simulink model "push_set_reset_Codegen"  (R2021a)
settings: Solver=FixedStepDiscrete  StartTime=0.0  StopTime=10  RelTol=1e-3
libraries: simulink x1
settings Model: Creator=surya  LastModifiedBy=surya
settings OptimizationCC: DefaultParameterBehavior=Inlined  EnhancedBackFolding=on  PassReuseOutputArgsAs=Individual arguments  ZeroExternalMemoryAtStartup=off  ZeroInternalMemoryAtStartup=off  OptimizeBlockOrder=speed  DifferentSizesBufferReuse=on  OptimizationCustomize=off  EfficientTunableParamExpr=on
settings DebuggingCC: ParameterTunabilityLossMsg=error
settings SFSimCC: MATLABDynamicMemAlloc=off
settings RTWCC: SystemTargetFile=ert.tlc  TemplateMakefile=ert_default_tmf
settings CodeAppCC: ForceParamTrailComments=on  IgnoreCustomStorageClasses=off  OperatorAnnotations=on  SimulinkDataObjDesc=on  SFDataObjDesc=on  InsertBlockDesc=on
settings ERTTargetCC: TargetLangStandard=C99 (ISO)  GenerateSampleERTMain=on  InlinedParameterPlacement=NonHierarchical  ERTCustomFileTemplate=example_file_process.tlc

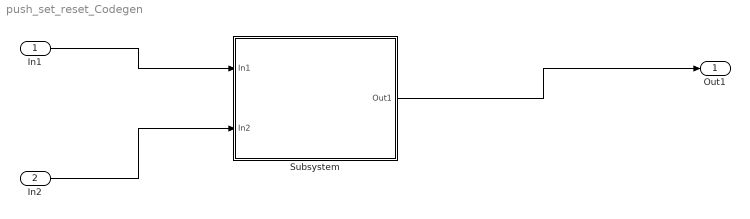
== system push_set_reset_Codegen ==
  In1 : Inport
  In2 : Inport  Port=2
  Subsystem : Subsystem  TreatAsAtomicUnit=on
  Out1 : Outport
  wires:
  In1/1 -> Subsystem/1(In1)
  In2/1 -> Subsystem/2(In2)
  Subsystem/1(Out1) -> Out1/1

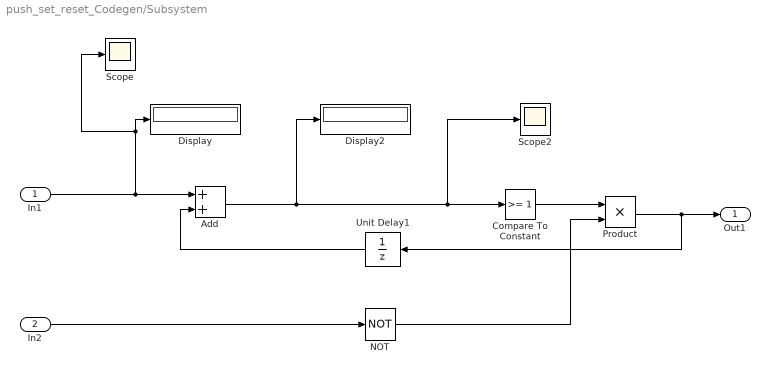
== system push_set_reset_Codegen/Subsystem ==
  In1 : Inport
  In2 : Inport  Port=2
  Add : Sum
  Compare To Constant : simulink/Logic and Bit Operations/Compare To Constant  relop=>=  const=1  OutDataTypeStr=boolean
  Display : Display
  Display2 : Display
  NOT : Logic  Operator=NOT  IconShape=distinctive  AllPortsSameDT=off  OutDataTypeStr=boolean
  Product : Product  OutDataTypeStr=double
  Scope : Scope
  Scope2 : Scope
  Unit Delay1 : UnitDelay  HasFrameUpgradeWarning=on
  Out1 : Outport
  wires:
  In1/1 -> Add/1, Display/1, Scope/1
  Product/1 -> Out1/1, Unit Delay1/1
  In2/1 -> NOT/1
  Unit Delay1/1 -> Add/2
  Add/1 -> Scope2/1, Compare To Constant/1, Display2/1
  NOT/1 -> Product/2
  Compare To Constant/1 -> Product/1
